simulink model "sistema_termico"  (R2025b)
settings: Solver=FixedStepAuto  StartTime=0.0  StopTime=inf  RelTol=1e-3  EnableMultiTasking=on
libraries: arduinolib x2
settings Model: ExtModeTrigDuration=2  Creator=Kleiton  LastModifiedBy=Kleiton
settings SolverCC: AutoInsertRateTranBlk=on
settings OptimizationCC: EnhancedBackFolding=on  PassReuseOutputArgsAs=Individual arguments  ZeroExternalMemoryAtStartup=off  ZeroInternalMemoryAtStartup=off  MaxStackSize=64  OptimizeBlockOrder=speed  DifferentSizesBufferReuse=on  OptimizationCustomize=off  EfficientTunableParamExpr=on
settings DebuggingCC: ParameterTunabilityLossMsg=error
settings HardwareCC: ProdBitPerInt=16.0  ProdBitPerPointer=16.0  ProdBitPerSizeT=16.0  ProdBitPerPtrDiffT=16.0  ProdLargestAtomicFloat=None  ProdWordSize=8.0  ProdHWDeviceType=Atmel->AVR
settings SFSimCC: MATLABDynamicMemAlloc=off
settings RTWCC: SystemTargetFile=ert.tlc  HardwareBoard=Arduino Uno  TemplateMakefile=ert_default_tmf  Toolchain=Arduino AVR  BuildConfiguration=Faster Runs  Description=Embedded Coder
settings CodeAppCC: ForceParamTrailComments=on  IgnoreCustomStorageClasses=off  OperatorAnnotations=on  SimulinkDataObjDesc=on  SFDataObjDesc=on  InsertBlockDesc=on
settings ERTTargetCC: ExtModeTransport=3.0  ExtModeStaticAlloc=on  ExtModeAutomaticAllocSize=off  ExtModeStaticAllocSize=250.0  ExtModeMexFile=ext_xcp  ExtModeIntrfLevel=Level2 - Open  InlinedParameterPlacement=Hierarchical  SupportContinuousTime=on  SupportVariableSizeSignals=on

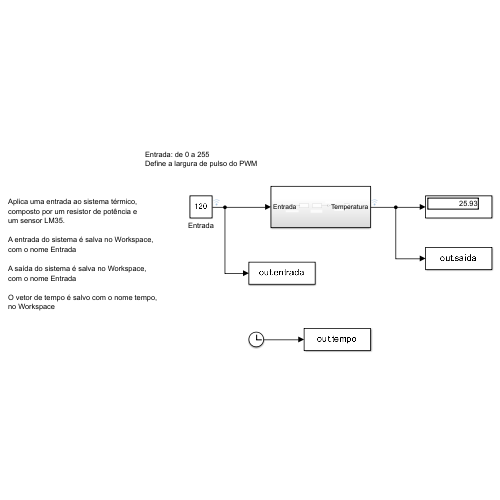
[thumbnail: Simulink's stored preview of the top-level diagram]
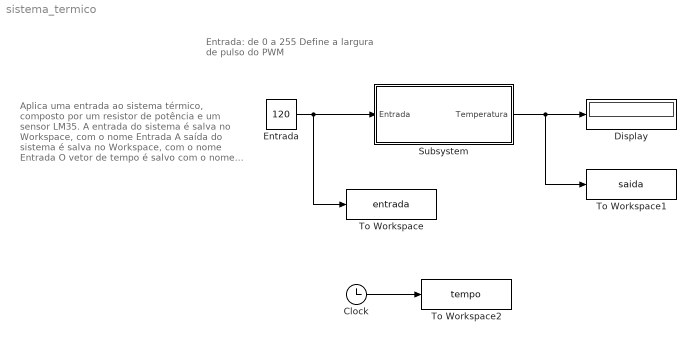
== system sistema_termico ==
  note: Aplica uma entrada ao sistema térmico,
      | composto por um resistor de potência e
      | um sensor LM35.
      |
      | A entrada do sistema é salva no Workspace,
      | com o nome Entrada
      |
      | A saída do sistema é salva no Workspace,
      | com o nome Entrada
      |
      | O vetor de tempo é salvo com o nome tempo,
      | no Workspace
  note: Entrada: de 0 a 255
      | Define a largura de pulso do PWM
  Clock : Clock
  Display : Display
  Entrada : Constant  Value=120
  Subsystem : Subsystem
  To Workspace : ToWorkspace  VariableName=entrada  SampleTime=-1
      settings: Save2DSignal=2-D array (concatenate along first dimension)
  To Workspace1 : ToWorkspace  VariableName=saida  SampleTime=-1
      settings: Save2DSignal=2-D array (concatenate along first dimension)
  To Workspace2 : ToWorkspace  VariableName=tempo  SampleTime=-1
      settings: Save2DSignal=2-D array (concatenate along first dimension)
  wires:
  Entrada/1 -> To Workspace/1, Subsystem/1(Entrada)
  Subsystem/1(Temperatura) -> To Workspace1/1, Display/1
  Clock/1 -> To Workspace2/1

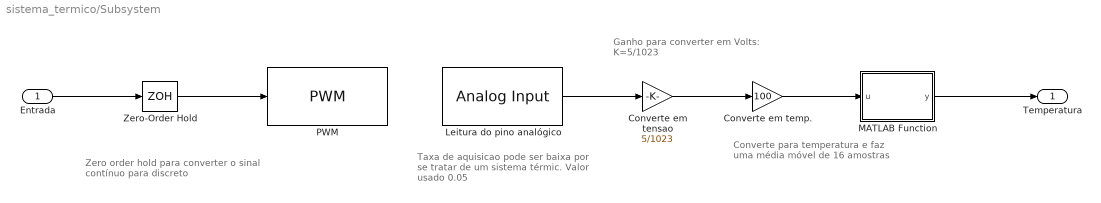
== system sistema_termico/Subsystem ==
  note: Zero order hold para converter o sinal
      | contínuo para discreto
  note: Ganho para converter em Volts:
      | K=5/1023
  note: Taxa de aquisicao pode ser baixa
      | por se tratar de um sistema térmic.
      | Valor usado 0.05
  note: Converte para temperatura e faz
      | uma média móvel de 16 amostras
  Entrada : Inport
  Converte em temp. : Gain  Gain=100  OutDataTypeStr=double
  Converte em tensao : Gain  Gain=5/1023  OutDataTypeStr=double
  Leitura do pino analógico : arduinolib/Analog Input  pinNumber=4  ReadResultsOnly=off  ConversionTriggerSource=Software  ExternalTriggerType=uint32( 0 )  OutputDataType=uint16  EnableConversionCompleteNotify=off  EnableOuputStatus=off  SampleTime=0.05  blockPlatform=arduino
  MATLAB Function : MATLAB Function  TreatAsAtomicUnit=on
  PWM : arduinolib/PWM  pinNumber=5  frequencyType=Default  desiredFrequency=200  achievableFrequency=490.2
  Zero-Order Hold : ZeroOrderHold  SampleTime=-1
  Temperatura : Outport
  wires:
  Zero-Order Hold/1 -> PWM/1
  Entrada/1 -> Zero-Order Hold/1
  Leitura do pino analógico/1 -> Converte em tensao/1
  Converte em tensao/1 -> Converte em temp./1
  Converte em temp./1 -> MATLAB Function/1(u)
  MATLAB Function/1(y) -> Temperatura/1

== matlab function sistema_termico/Subsystem/MATLAB Function ==
  data: u input; y output
function y = fcn(u)
    N = 32; % Número de amostras da média móvel
    
    persistent buffer count
    if isempty(buffer)
        buffer = zeros(1, N);
        count = 0;
    end

    % Atualiza o histórico (Fila FIFO)
    buffer = [buffer(2:end), u];
    
    % Incrementa a contagem de amostras recebidas
    if count < N
        count = count + 1;
    end

    % Calcula a média móvel das amostras válidas
    y = sum(buffer(end-count+1:end)) / count;
end
